simulink model "sae_j1772"  (R2024a)
settings: Solver=VariableStepAuto  StartTime=0.0  StopTime=10.0  RelTol=1e-3
InitFcn:
  | PilotVolt = single(5);
  | ProxVolt = single(1.5);
  | DutyCycle = single(0.1);
  | VehOk = logical(true);
  | BattCurr = single(-0.2);
libraries: autolibevcharging x1
settings Model: PacingRate=0.100000  Creator=jh2beauty  LastModifiedBy=jh2beauty

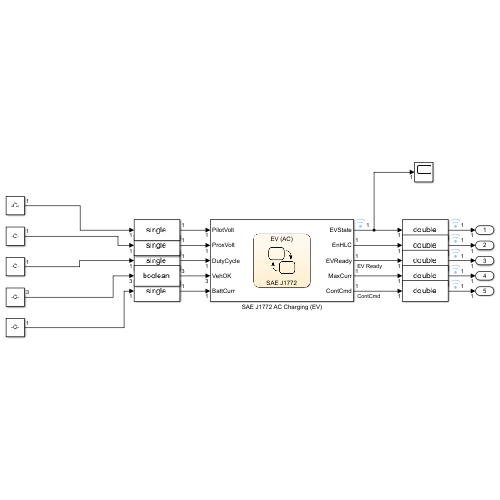
[thumbnail: Simulink's stored preview of the top-level diagram]
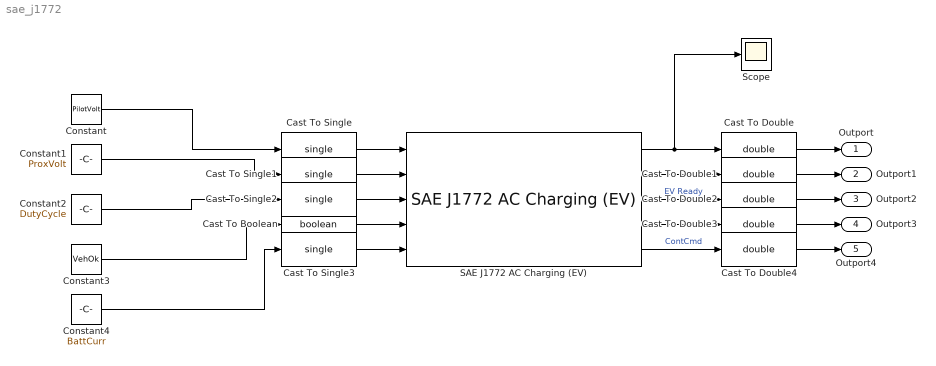
== system sae_j1772 ==
  Cast To Boolean : DataTypeConversion  OutDataTypeStr=boolean  SaturateOnIntegerOverflow=off  RndMeth=Floor
  Cast To Double{,1..4} (5 alike) : DataTypeConversion  OutDataTypeStr=double  SaturateOnIntegerOverflow=off  RndMeth=Floor
  Cast To Single{,1..3} (4 alike) : DataTypeConversion  OutDataTypeStr=single  SaturateOnIntegerOverflow=off  RndMeth=Floor
  Constant : Constant  Value=PilotVolt
  Constant1 : Constant  Value=ProxVolt
  Constant2 : Constant  Value=DutyCycle
  Constant3 : Constant  Value=VehOk
  Constant4 : Constant  Value=BattCurr
  SAE J1772 AC Charging (EV) : autolibevcharging/SAE J1772 AC Charging (EV)  T_contactor_delay=3  Ts=0.1  aMode=1
  Scope : Scope
  Outport : Outport
  Outport1 : Outport  Port=2
  Outport2 : Outport  Port=3
  Outport3 : Outport  Port=4
  Outport4 : Outport  Port=5
  wires:
  SAE J1772 AC Charging (EV)/5 -> Cast To Double4/1  "ContCmd"
  SAE J1772 AC Charging (EV)/4 -> Cast To Double3/1
  SAE J1772 AC Charging (EV)/3 -> Cast To Double2/1  "EV Ready"
  SAE J1772 AC Charging (EV)/2 -> Cast To Double1/1
  SAE J1772 AC Charging (EV)/1 -> Scope/1, Cast To Double/1
  Cast To Double/1 -> Outport/1
  Cast To Double1/1 -> Outport1/1
  Cast To Double2/1 -> Outport2/1
  Cast To Double3/1 -> Outport3/1
  Cast To Double4/1 -> Outport4/1
  Constant/1 -> Cast To Single/1
  Cast To Single/1 -> SAE J1772 AC Charging (EV)/1
  Cast To Single1/1 -> SAE J1772 AC Charging (EV)/2
  Cast To Single2/1 -> SAE J1772 AC Charging (EV)/3
  Cast To Single3/1 -> SAE J1772 AC Charging (EV)/5
  Cast To Boolean/1 -> SAE J1772 AC Charging (EV)/4
  Constant1/1 -> Cast To Single1/1
  Constant2/1 -> Cast To Single2/1
  Constant3/1 -> Cast To Boolean/1
  Constant4/1 -> Cast To Single3/1
